simulink model "Pub_Sub_Husqvarna"  (R2017a)
settings: Solver=VariableStepAuto  StartTime=0.0  StopTime=inf  RelTol=1e-3
undefined symbols (not defined in the file): LinearAcceleration
libraries: robotlib x2, fuzblock x1
settings Model: Creator=francesco  LastModifiedBy=francesco

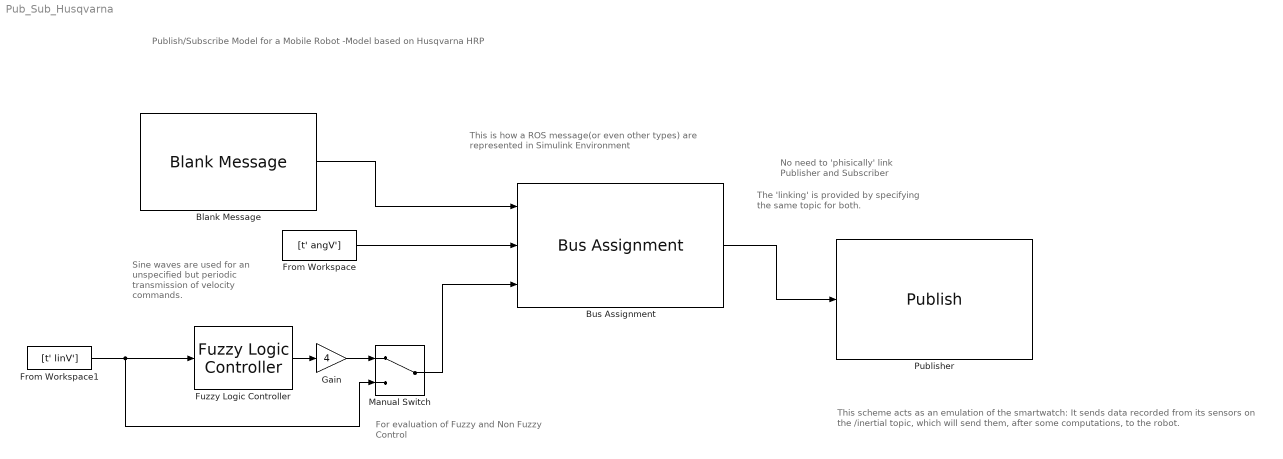
== system Pub_Sub_Husqvarna ==
  note: This scheme acts as an emulation of the smartwatch:
      | It sends data recorded from its sensors on the /inertial
      | topic, which will send them, after some computations, to the robot.
  note: For evaluation of Fuzzy and Non Fuzzy
      | Control
  note: This is how a ROS message(or even other types)
      |  are represented in Simulink Environment
  note: Sine waves are used for an
      | unspecified but periodic
      | transmission of velocity
      | commands.
  note: Publish/Subscribe Model for a Mobile Robot
      | -Model based on Husqvarna HRP
  note: No need to 'phisically' link
      | Publisher and Subscriber
  note: The 'linking' is provided by specifying
      | the same topic for both.
  Blank Message : robotlib/Blank Message  SourceLibraryInfo=This block requires Robotics System Toolbox  messageType=sensor_msgs/Imu  SampleTime=inf
      settings: SourceProductBaseCode=RO
  Bus Assignment : BusAssignment  AssignedSignals=LinearAcceleration.Z,LinearAcceleration.X
  From Workspace : FromWorkspace  VariableName=[t' angV']  OutDataTypeStr=double  SampleTime=0  Interpolate=off  OutputAfterFinalValue=Setting to zero
  From Workspace1 : FromWorkspace  VariableName=[t' linV']  OutDataTypeStr=double  SampleTime=0  Interpolate=off  OutputAfterFinalValue=Setting to zero
  Fuzzy Logic Controller : fuzblock/Fuzzy Logic  Controller  fis='LinVelDefinitivo.fis'
  Gain : Gain  Gain=4
  Manual Switch : ManualSwitch
  Publisher : robotlib/Publish  SourceLibraryInfo=This block requires Robotics System Toolbox  topicSource=Select from ROS network  topic=/inertial  messageType=sensor_msgs/Imu  messageQueueLength=1
      settings: SourceProductBaseCode=RO
  wires:
  Bus Assignment/1 -> Publisher/1
  From Workspace1/1 -> Manual Switch/2, Fuzzy Logic Controller/1
  From Workspace/1 -> Bus Assignment/2
  Manual Switch/1 -> Bus Assignment/3
  Blank Message/1 -> Bus Assignment/1
  Fuzzy Logic Controller/1 -> Gain/1
  Gain/1 -> Manual Switch/1
